simulink model "ARbotTemplate"  (R2019b)
settings: Solver=VariableStepAuto  StartTime=0.0  StopTime=inf  RelTol=1e-3
PreLoadFcn:
  | % ROS setup
  | clear all;
  | clc;
  | 
  | 
  | %
  | 
  | setenv('CUDA_PATH',fullfile("C:","Program Files","NVIDIA GPU Computing Toolkit","CUDA","v10.1"))
  | setenv('NVIDIA_CUDNN',fullfile("C:","Program Files","NVIDIA GPU Computing Toolkit","CUDA","cuDNN"));
  | setenv('NVIDIA_TENSORRT', fullfile("C:","Program Files","NVIDIA GPU Computing Toolkit","CUDA","TensorRT"))
  | setenv('OPENCV_DIR',fullfile("C:","Program Files","opencv","build"));
  | setenv('PATH', ...
  |     [fullfile('C:','Program Files','NVIDIA GPU Computing Toolkit','CUDA','v10.1','bin') ';' ...
  |     fullfile('C:','Program Files','NVIDIA GPU Computing Toolkit','CUDA','cuDNN','bin') ';'...
  |     fullfile('C:','Program Files','opencv','build','x64','vc15','bin') ';'...
  |     fullfile('C:','Program Files','NVIDIA GPU Computing Toolkit','CUDA','TensorRT','lib') ';'...
  |     getenv('PATH')]);
  | 
  | run('preload_ARbot_Script_Deploy_v1.m');
  | 
  | % Sample times
  | sampleTime = 0.2;
  | 
  | % Control parameters
  | ctrlParam1 = 2;
  | ctrlParam2 = 3.5;
undefined symbols (not defined in the file or in its folder): X, Y
libraries: robotlib x2, visionsources x1
settings Model: Creator=scastro  LastModifiedBy=Visitor
settings DataIOCC: ReturnWorkspaceOutputs=off
settings DebuggingCC: ArithmeticOperatorsInVariantConditions=warning
settings SFSimCC: SimUseLocalCustomCode=off  CustomCodeUndefinedFunction=UseInterfaceOnly
settings RTWCC: RTWUseLocalCustomCode=off

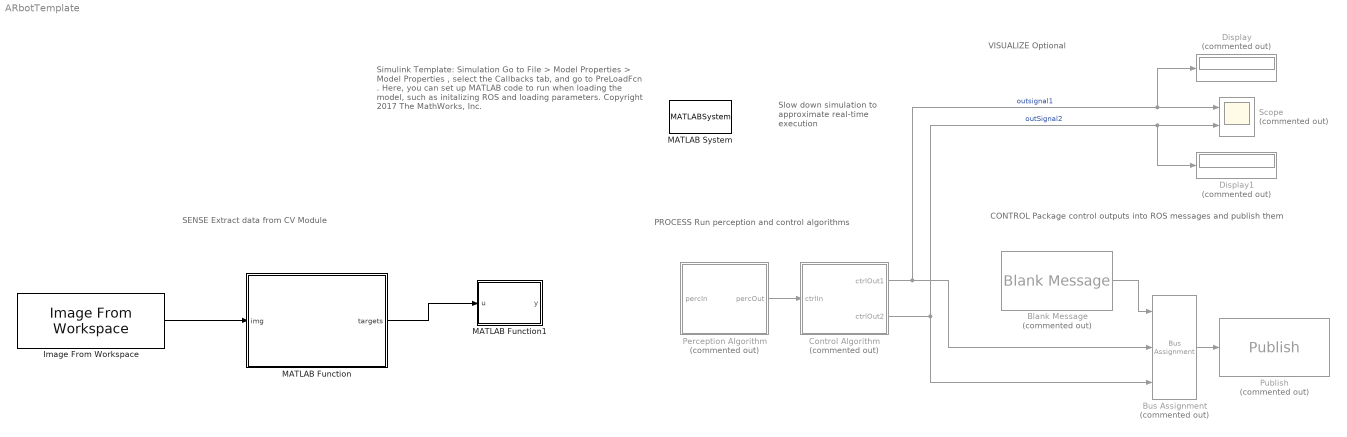
== system ARbotTemplate ==
  note: Simulink Template: Simulation
      |
      | Go to File > Model Properties > Model Properties , select the Callbacks tab, and go to PreLoadFcn .
      |
      | Here, you can set up MATLAB code to run when loading the model, such as initalizing ROS and loading parameters.
      |
      | Copyright 2017 The MathWorks, Inc.
  note: Slow down simulation to approximate real-time execution
  note: PROCESS
      | Run perception and control algorithms
  note: SENSE
      | Extract data from CV Module
  note: VISUALIZE
      | Optional
  note: CONTROL
      | Package control outputs into ROS messages and publish them
  Blank Message : robotlib/Blank Message  Commented=on  messageClass=Message  entityType=geometry_msgs/Point  messageType=geometry_msgs/Point  SampleTime=inf
      settings: SourceProductBaseCode=RO
  Bus Assignment : BusAssignment  Commented=on  AssignedSignals=X,Y
  Control Algorithm : Subsystem  Commented=on
  Display : Display  Commented=on
  Display1 : Display  Commented=on
  Image From Workspace : visionsources/Image From Workspace  Tag=vipblks_nd  ImageValue=inImg  Ts=inf  imagePorts=One multidimensional signal  OutPortLabels=R|G|B  ImageDataType=Inherit from 'Value'  Signed=on  WordLength=16  sdImageDataType=sfix(16)  FractionLengthMode=User-defined  FractionLength=15
      settings: SourceProductName=Computer Vision Toolbox  SourceProductBaseCode=VP
  MATLAB Function : MATLAB Function  TreatAsAtomicUnit=on
  MATLAB Function1 : MATLAB Function  TreatAsAtomicUnit=on
  MATLAB System : MATLABSystem  System=ExampleHelperSimulationRateControl  SampleTime=0.2
      mask Type: ExampleHelperSimulationRateControl
      mask Display: disp('Rate Control');
  Perception Algorithm : Subsystem  Commented=on
  Publish : robotlib/Publish  Commented=on  topicSource=Specify your own  topic=/my_pub_topic  messageType=geometry_msgs/Point  messageQueueLength=1
      settings: SourceProductBaseCode=RO
  Scope : Scope  Commented=on  NumInputPorts=2
  wires:
  Bus Assignment/1 -> Publish/1
  Blank Message/1 -> Bus Assignment/1
  Perception Algorithm/1(percOut) -> Control Algorithm/1(ctrlIn)
  Control Algorithm/1(ctrlOut1) -> Bus Assignment/2, Display/1, Scope/1  "outsignal1"
  Control Algorithm/2(ctrlOut2) -> Display1/1, Scope/2, Bus Assignment/3  "outSignal2"
  Image From Workspace/1 -> MATLAB Function/1(img)
  MATLAB Function/1(targets) -> MATLAB Function1/1(u)

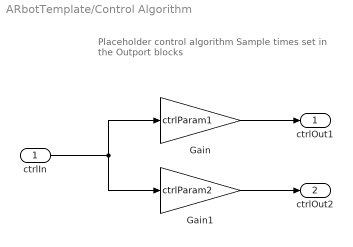
== system ARbotTemplate/Control Algorithm ==
  note: Placeholder control algorithm
      |
      | Sample times set in the Outport blocks
  ctrlIn : Inport
  Gain : Gain  Gain=ctrlParam1
  Gain1 : Gain  Gain=ctrlParam2
  ctrlOut1 : Outport  SampleTime=sampleTime  VectorParamsAs1DForOutWhenUnconnected=off
      settings: AttributesFormatString=Sample time: %<SampleTime>
  ctrlOut2 : Outport  Port=2  SampleTime=sampleTime  VectorParamsAs1DForOutWhenUnconnected=off
      settings: AttributesFormatString=Sample time: %<SampleTime>
  wires:
  ctrlIn/1 -> Gain1/1, Gain/1
  Gain/1 -> ctrlOut1/1
  Gain1/1 -> ctrlOut2/1

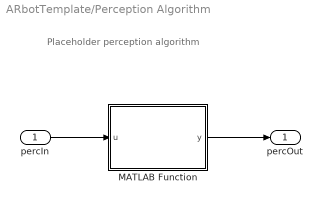
== system ARbotTemplate/Perception Algorithm ==
  note: Placeholder perception algorithm
  percIn : Inport
  MATLAB Function : MATLAB Function  TreatAsAtomicUnit=on
  percOut : Outport  VectorParamsAs1DForOutWhenUnconnected=off
  wires:
  percIn/1 -> MATLAB Function/1(u)
  MATLAB Function/1(y) -> percOut/1

== matlab function ARbotTemplate/MATLAB Function ==
  data: targets output; total_Targets_Possible parameter; img input
function targets = roboSubPredictSimulink(total_Targets_Possible, img)
%#codegen

%hwobj = jetson;
%w = webcam(hwobj,1);
%d = imageDisplay(hwobj);

targets = 0;
bboxMat = zeros(total_Targets_Possible,4);
persistent yolo2Object;
if isempty(yolo2Object)
    yolo2Object = coder.loadDeepLearningNetwork('resnet101_10_preprocessed.mat');
    % yolo2Object = load('resnet101_10_preprocessed.mat');
end
% grab an image and annotate it
img = imresize(img,[224 224]);
[bboxes,scores,labels] = yolo2Object.detect(img,'Threshold',0.6);
% %[bboxes,scores] = detect(yolo2Object.detector,img);
% [~,idx] = max(scores);
% 
% bboxesSize = size(bboxes);
% 
% for i=1:bboxesSize(1)
%     for j = 1:4
%         bboxMat(i,j) = bboxes(i,j); 
%     end
% end
% 
% % Annotate detections in the image.
% if ~isempty(bboxes)
%     outImg = insertObjectAnnotation(img,'Rectangle',bboxes(idx,:),labels{idx});
% else
%     outImg = img;
% end
% imshow(outImg);
% 
% targets = 4;

end

== matlab function ARbotTemplate/Perception Algorithm/MATLAB Function ==
  data: u input; y output
function y = myPerceptionFcn(u)

y = 2*u;

== matlab function ARbotTemplate/MATLAB Function1 ==
  data: u input; y output
function y = fcn(u)

y = u;
